simulink model "Suspension"  (R2019b)
settings: Solver=VariableStepAuto  StartTime=0.0  StopTime=10.0  RelTol=1e-3
values from neighbouring files (symbols this model uses):
  Cf = 2500    [Suspension_Datas.m]    (also in matlab_suspensiondata.mat)
  Cr = 2000    [Suspension_Datas.m]    (also in matlab_suspensiondata.mat)
  Iyy = 2100    [Suspension_Datas.m]    (also in matlab_suspensiondata.mat)
  Kf = 1    [ABS_Datas.m]    (also in Suspension_Datas.m = 28000; matlab_ABSdata.mat; matlab_suspensiondata.mat = 28000)
  Kr = 21000    [Suspension_Datas.m]    (also in matlab_suspensiondata.mat)
  Lf = 0.9    [Suspension_Datas.m]    (also in matlab_suspensiondata.mat)
  Lr = 1.2    [Suspension_Datas.m]    (also in matlab_suspensiondata.mat)
  mb = 1200    [Suspension_Datas.m]    (also in matlab_suspensiondata.mat)
settings Model: Creator=Yogesh  LastModifiedBy=Tharun

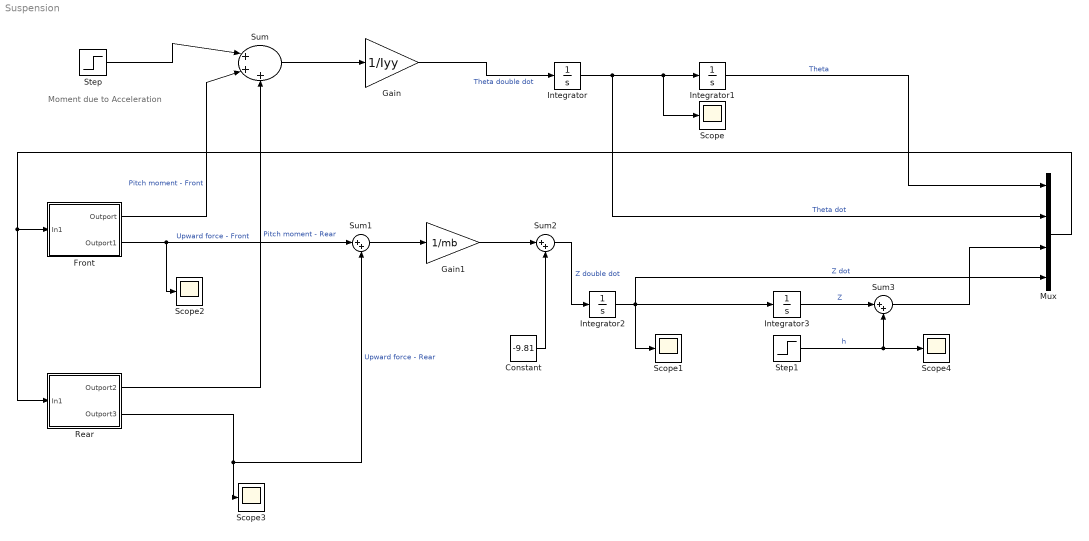
== system Suspension ==
  note: Moment due to Acceleration
  Constant : Constant  Value=-9.81
  Front : Subsystem
  Gain : Gain  Gain=1/Iyy
  Gain1 : Gain  Gain=1/mb
  Integrator{,1..3} (4 alike) : Integrator
  Mux : Mux
  Rear : Subsystem
  Scope{,1..4} (5 alike) : Scope
  Step : Step  Time=3  After=1000  SampleTime=0
  Step1 : Step  Time=7  After=5  SampleTime=0
  Sum : Sum  Inputs=|+++
  Sum1 : Sum  Inputs=|++
  Sum2 : Sum  Inputs=|++
  Sum3 : Sum  Inputs=|++
  wires:
  Step/1 -> Sum/1
  Rear/1(Outport2) -> Sum/3  "Pitch moment - Rear"
  Front/1(Outport) -> Sum/2  "Pitch moment - Front"
  Sum/1 -> Gain/1
  Gain/1 -> Integrator/1  "Theta double dot"
  Integrator/1 -> Mux/2, Scope/1, Integrator1/1  "Theta dot"
  Integrator1/1 -> Mux/1  "Theta"
  Front/2(Outport1) -> Scope2/1, Sum1/1  "Upward force - Front"
  Rear/2(Outport3) -> Sum1/2, Scope3/1  "Upward force - Rear"
  Sum1/1 -> Gain1/1
  Gain1/1 -> Sum2/1
  Sum2/1 -> Integrator2/1  "Z double dot"
  Integrator2/1 -> Scope1/1, Mux/4, Integrator3/1  "Z dot"
  Integrator3/1 -> Sum3/1  "Z"
  Step1/1 -> Scope4/1, Sum3/2  "h"
  Sum3/1 -> Mux/3
  Mux/1 -> Front/1(In1), Rear/1(In1)
  Constant/1 -> Sum2/2

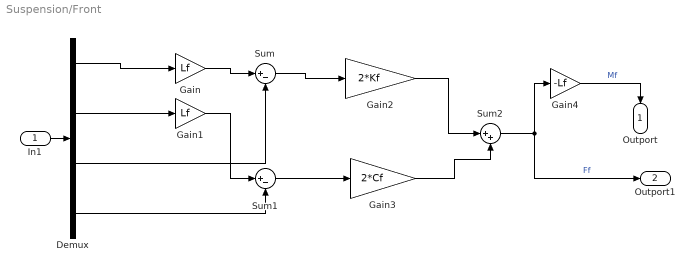
== system Suspension/Front ==
  In1 : Inport
  Demux : Demux
  Gain : Gain  Gain=Lf
  Gain1 : Gain  Gain=Lf
  Gain2 : Gain  Gain=2*Kf
  Gain3 : Gain  Gain=2*Cf
  Gain4 : Gain  Gain=-Lf
  Sum : Sum  Inputs=|+-
  Sum1 : Sum  Inputs=|+-
  Sum2 : Sum  Inputs=|++
  Outport : Outport
  Outport1 : Outport  Port=2
  wires:
  Sum1/1 -> Gain3/1
  Sum2/1 -> Outport1/1, Gain4/1  "Ff"
  Sum/1 -> Gain2/1
  Gain4/1 -> Outport/1  "Mf"
  Demux/2 -> Gain1/1
  Demux/4 -> Sum1/2
  Gain3/1 -> Sum2/2
  Gain2/1 -> Sum2/1
  Gain1/1 -> Sum1/1
  Demux/3 -> Sum/2
  In1/1 -> Demux/1
  Demux/1 -> Gain/1
  Gain/1 -> Sum/1

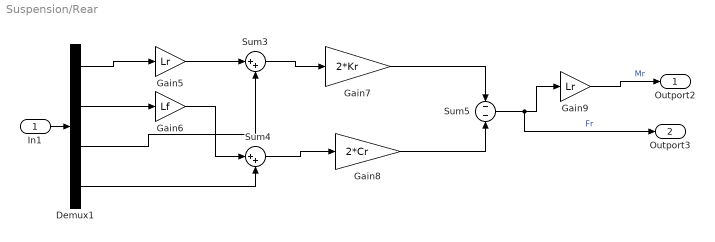
== system Suspension/Rear ==
  In1 : Inport
  Demux1 : Demux
  Gain5 : Gain  Gain=Lr
  Gain6 : Gain  Gain=Lf
  Gain7 : Gain  Gain=2*Kr
  Gain8 : Gain  Gain=2*Cr
  Gain9 : Gain  Gain=Lr
  Sum3 : Sum  Inputs=|++
  Sum4 : Sum  Inputs=|++
  Sum5 : Sum  Inputs=--
  Outport2 : Outport
  Outport3 : Outport  Port=2
  wires:
  Sum5/1 -> Outport3/1, Gain9/1  "Fr"
  Demux1/1 -> Gain5/1
  Gain5/1 -> Sum3/1
  Gain8/1 -> Sum5/2
  Gain6/1 -> Sum4/1
  Demux1/3 -> Sum3/2
  Gain7/1 -> Sum5/1
  Demux1/4 -> Sum4/2
  Sum4/1 -> Gain8/1
  Gain9/1 -> Outport2/1  "Mr"
  In1/1 -> Demux1/1
  Sum3/1 -> Gain7/1
  Demux1/2 -> Gain6/1
